simulink model "Pr4"  (R2022b)
settings: Solver=ode23  StartTime=0.0  StopTime=600  RelTol=1e-3
libraries: simulink x1
settings Model: Creator=rus_d  LastModifiedBy=rus_d

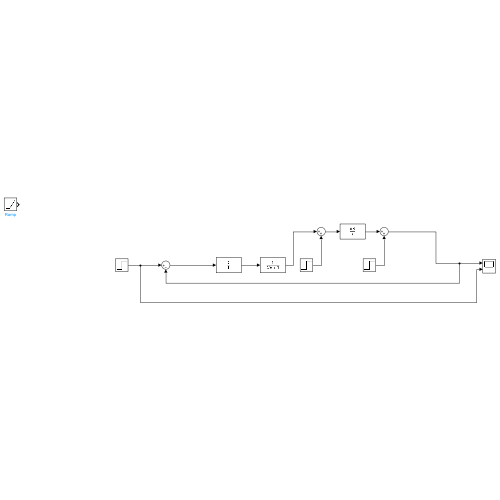
[thumbnail: Simulink's stored preview of the top-level diagram]
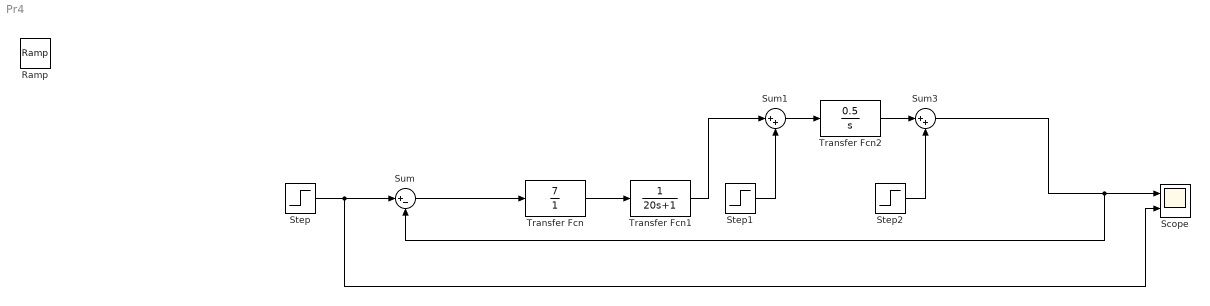
== system Pr4 ==
  Ramp : simulink/Sources/Ramp  slope=1  start=0  InitialOutput=0
  Scope : Scope  NumInputPorts=2
  Step : Step  SampleTime=0
  Step1 : Step  Time=200  After=0.2  SampleTime=0
  Step2 : Step  Time=400  After=0.1  SampleTime=0
  Sum : Sum  Inputs=|+-
  Sum1 : Sum  Inputs=|++
  Sum3 : Sum  Inputs=|++
  Transfer Fcn : TransferFcn  Numerator=[7]  Denominator=[1]
  Transfer Fcn1 : TransferFcn  Denominator=[20 1]
  Transfer Fcn2 : TransferFcn  Numerator=[0.5]  Denominator=[1 0]
  wires:
  Step2/1 -> Sum3/2
  Sum/1 -> Transfer Fcn/1
  Transfer Fcn/1 -> Transfer Fcn1/1
  Step1/1 -> Sum1/2
  Transfer Fcn1/1 -> Sum1/1
  Sum1/1 -> Transfer Fcn2/1
  Transfer Fcn2/1 -> Sum3/1
  Sum3/1 -> Sum/2, Scope/1
  Step/1 -> Scope/2, Sum/1
